simulink model "external_jarmu"  (R2018b)
settings: Solver=ode3  StartTime=0.0  StopTime=inf  FixedStep=0.01  RelTol=1e-3
model workspace (MAT data in the model file):
  CdA = Simulink.Parameter
  CdA.Value = 0.576
  CdA.DataType = 'auto'
  CdA.Dimensions = [1 1]
  g = Simulink.Parameter
  g.Value = 9.81
  g.DataType = 'auto'
  g.Dimensions = [1 1]
  m = Simulink.Parameter
  m.Value = 2200
  m.DataType = 'auto'
  m.Dimensions = [1 1]
  p = Simulink.Parameter
  p.Value = 1.2
  p.DataType = 'auto'
  p.Dimensions = [1 1]
  v = Simulink.Parameter
  v.DataType = 'auto'
  v.Dimensions = [0 0]
libraries: retelab_lib x2, simulink_extras x1
settings Model: SimulationMode=external  Creator=cloud  LastModifiedBy=cloud
settings RTWCC: SystemTargetFile=sldrt.tlc  TemplateMakefile=sldrt.tmf  Description=Simulink Desktop Real-Time  RTWCompilerOptimization=on
settings CodeAppCC: MaxIdLength=95
settings SimulinkDesktopRealTimeCC: TargetPreCompLibLocation=C:\Program Files\MATLAB\R2018a\toolbox\sldrt\lib\win64  PreserveStateflowLocalDataDimensions=off

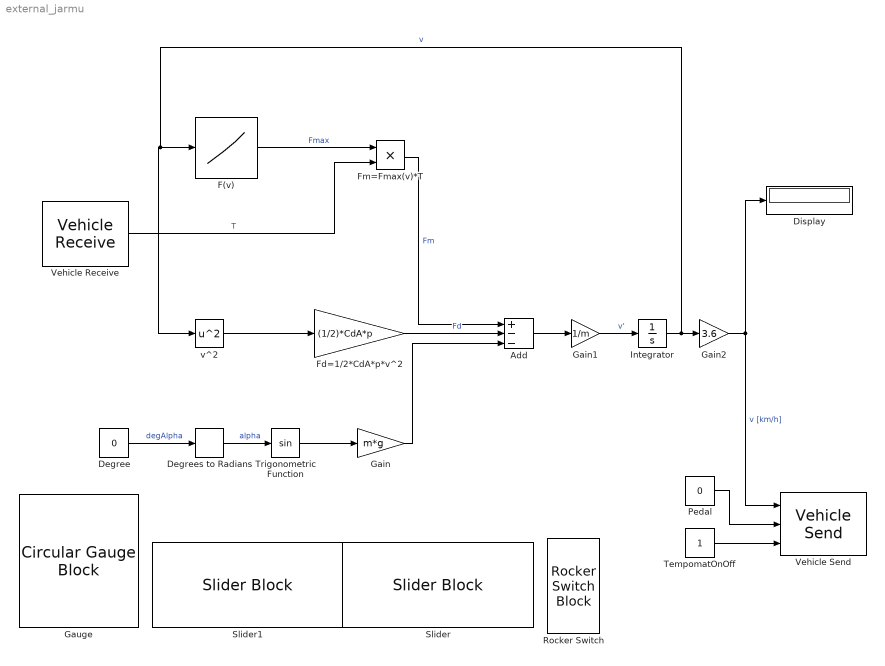
== system external_jarmu ==
  Add : Sum  Inputs=+--
  Degree : Constant  Value=0
  Degrees to Radians : simulink_extras/Transformations/Degrees to Radians
  Display : Display
  F(v) : Lookup_n-D  NumberOfTableDimensions=1  BreakpointsForDimension1=[20 27 36 53]  Table=[14500 7200 3800 1900]  InterpMethod=Cubic spline  ExtrapMethod=Clip  InternalRulePriority=Speed  RndMeth=Simplest  InputSameDT=on
  Fd=1/2*CdA*p*v^2 : Gain  Gain=(1/2)*CdA*p
  Fm=Fmax(v)*T : Product
  Gain : Gain  Gain=m*g
  Gain1 : Gain  Gain=1/m
  Gain2 : Gain  Gain=3.6
  Gauge : CircularGaugeBlock  WebBlockId=23  ScaleMax=260
  Integrator : Integrator  InitialCondition=37  LimitOutput=on  UpperSaturationLimit=100  LowerSaturationLimit=0
  Pedal : Constant  Value=0
  Rocker Switch : RockerSwitchBlock  WebBlockId=18
      settings: Values={{'Off', 'On'}, [0 1]}
  Slider : SliderBlock  WebBlockId=19  ScaleMax=1
  Slider1 : SliderBlock  WebBlockId=20  ScaleMax=10
  TempomatOnOff : Constant
  Trigonometric Function : Trigonometry
  Vehicle Receive : retelab_lib/Vehicle Receive  SystemSampleTime=-1
      settings: SourceProductName=IIT1
  Vehicle Send : retelab_lib/Vehicle Send  SystemSampleTime=-1
      settings: SourceProductName=IIT1
  v^2 : Math  Operator=square  SaturateOnIntegerOverflow=on
  wires:
  Add/1 -> Gain1/1
  Integrator/1 -> v^2/1, F(v)/1, Gain2/1  "v"
  Gain1/1 -> Integrator/1  "v'"
  v^2/1 -> Fd=1/2*CdA*p*v^2/1
  Gain/1 -> Add/3
  Gain2/1 -> Display/1, Vehicle Send/1  "v [km/h]"
  F(v)/1 -> Fm=Fmax(v)*T/1  "Fmax"
  Degrees to Radians/1 -> Trigonometric Function/1  "alpha"
  Trigonometric Function/1 -> Gain/1
  Fm=Fmax(v)*T/1 -> Add/1  "Fm"
  Fd=1/2*CdA*p*v^2/1 -> Add/2  "Fd"
  Vehicle Receive/1 -> Fm=Fmax(v)*T/2  "T"
  Degree/1 -> Degrees to Radians/1  "degAlpha"
  TempomatOnOff/1 -> Vehicle Send/3
  Pedal/1 -> Vehicle Send/2
